simulink model "step_4"  (R2020a)
settings: Solver=VariableStepAuto  StartTime=0.0  StopTime=10.0  RelTol=1e-3
settings Model: Creator=HP  LastModifiedBy=HP

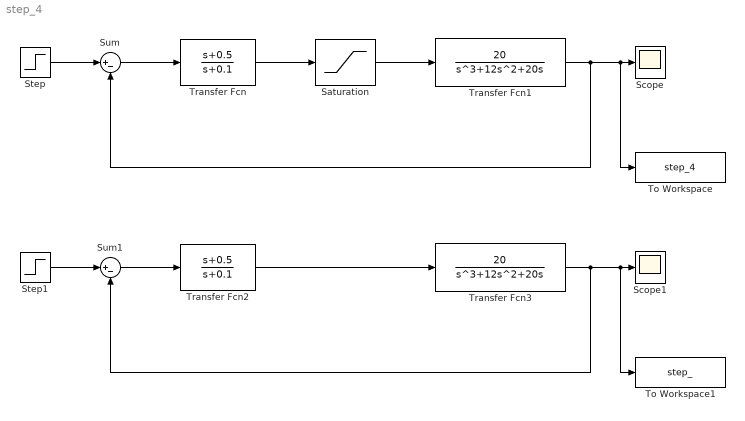
== system step_4 ==
  Saturation : Saturate  UpperLimit=5  LowerLimit=-5
  Scope : Scope
  Scope1 : Scope
  Step : Step  Time=0  After=10  SampleTime=0
  Step1 : Step  Time=0  After=10  SampleTime=0
  Sum : Sum  Inputs=|+-
  Sum1 : Sum  Inputs=|+-
  To Workspace : ToWorkspace  VariableName=step_4  SampleTime=0.001
  To Workspace1 : ToWorkspace  VariableName=step_  SampleTime=0.001
  Transfer Fcn : TransferFcn  Numerator=[1 0.5]  Denominator=[1 0.1]
  Transfer Fcn1 : TransferFcn  Numerator=[20]  Denominator=[1 12 20 0]
  Transfer Fcn2 : TransferFcn  Numerator=[1 0.5]  Denominator=[1 0.1]
  Transfer Fcn3 : TransferFcn  Numerator=[20]  Denominator=[1 12 20 0]
  wires:
  Sum/1 -> Transfer Fcn/1
  Step/1 -> Sum/1
  Transfer Fcn/1 -> Saturation/1
  Saturation/1 -> Transfer Fcn1/1
  Transfer Fcn1/1 -> Sum/2, To Workspace/1, Scope/1
  Transfer Fcn2/1 -> Transfer Fcn3/1
  Sum1/1 -> Transfer Fcn2/1
  Step1/1 -> Sum1/1
  Transfer Fcn3/1 -> Sum1/2, To Workspace1/1, Scope1/1
